simulink model "series_blance_leg"  (R2022b)
settings: Solver=ode45  StartTime=0.0  StopTime=10  MaxStep=0.2  RelTol=1e-3
values from neighbouring files (symbols this model uses):
  a11 = polyfit(leg,k11,3)    [series_get_k.m]
  a12 = polyfit(leg,k12,3)    [series_get_k.m]
  a13 = polyfit(leg,k13,3)    [series_get_k.m]
  a14 = polyfit(leg,k14,3)    [series_get_k.m]
  a15 = polyfit(leg,k15,3)    [series_get_k.m]
  a16 = polyfit(leg,k16,3)    [series_get_k.m]
  a21 = polyfit(leg,k21,3)    [series_get_k.m]
  a22 = polyfit(leg,k22,3)    [series_get_k.m]
  a23 = polyfit(leg,k23,3)    [series_get_k.m]
  a24 = polyfit(leg,k24,3)    [series_get_k.m]
  a25 = polyfit(leg,k25,3)    [series_get_k.m]
  a26 = polyfit(leg,k26,3)    [series_get_k.m]
  N = NM + mp*diff(x + L*sin(theta),t,2)    [series_get_k_length.m]
undefined symbols (not defined in the file or in its folder): X, Y, Z
libraries: sm_lib x60, nesl_utility x20, matrix_library x8, slpidlib x2, cstblocks x2
(part 1 of 3)
settings Model: SimulationMode=accelerator  Creator=Hhop  LastModifiedBy=admin
settings SolverCC: MinimalZcImpactIntegration=on
settings DataIOCC: ReturnWorkspaceOutputs=off
settings DebuggingCC: ReadBeforeWriteMsg=DisableAll  WriteAfterWriteMsg=DisableAll  WriteAfterReadMsg=DisableAll  MultiTaskDSMMsg=none
settings ModelReferenceCC: UpdateModelReferenceTargets=IfOutOfDate
settings SFSimCC: SFSimEcho=off

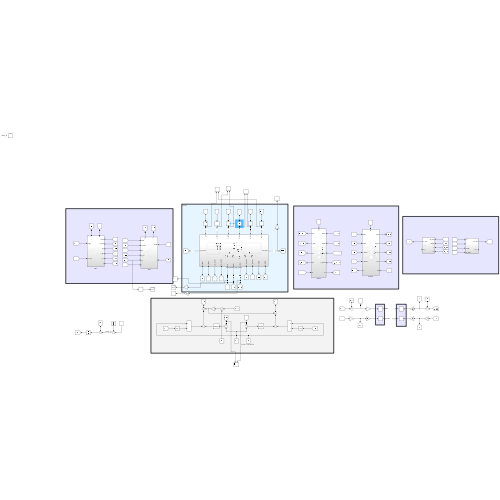
[thumbnail: Simulink's stored preview of the top-level diagram]
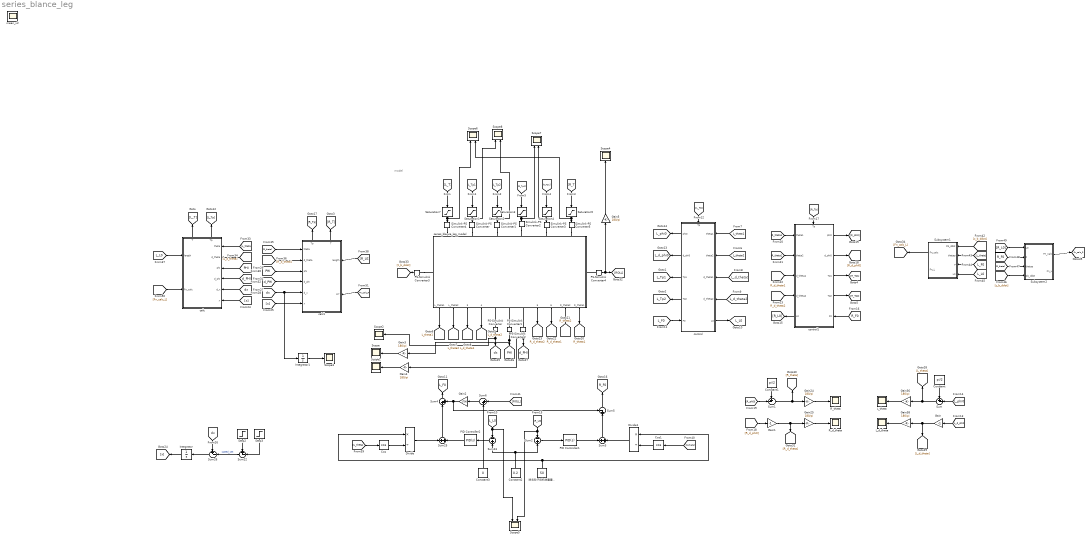
== system series_blance_leg ==
  note: model
  Constant : Constant  Value=pi/2
  Constant1 : Constant  Value=pi/2
  Constant2 : Constant  Value=0.2
  Constant3 : Constant  Value=0
  Cos : Trigonometry  Operator=cos
  Cos1 : Trigonometry  Operator=cos
  Divide : Product  Inputs=*/
  Divide1 : Product  Inputs=*/
  Gain : Gain  Gain=-1
  Gain1 : Gain  Gain=-1
  Gain2 : Gain  Gain=1700
  Gain{3..5,24..25,36,38} (7 alike) : Gain  Gain=180/pi
  Integrator : Integrator
  Integrator1 : Integrator
  L_d_theta : Scope
  L_theta : Scope
  PID Controller1 : slpidlib/PID Controller  Controller=PID  Form=Parallel  TimeDomain=Continuous-time  UseExternalTs=off  SampleTime=-1  IntegratorMethod=Forward Euler  FilterMethod=Forward Euler  ControllerParametersSource=internal  P=800  I=0  UseKiTs=off  D=300  N=100  UseFilter=on  TunerSelectOption=Transfer Function Based (PID Tuner App)  InitialConditionSource=internal  InitialConditionForIntegrator=0  InitialConditionForFilter=0  DifferentiatorICPrevScaledInput=0  ExternalReset=none  TrackingMode=off  Kt=1  LimitOutput=off  SatLimitsSource=internal  UpperSaturationLimit=inf  LowerSaturationLimit=-inf  LinearizeAsGain=on  AntiWindupMode=none  Kb=1  LimitIntegrator=off  UpperIntegratorSaturationLimit=inf  LowerIntegratorSaturationLimit=-inf  POutMin=[]  POutMax=[]  IOutMin=[]  IOutMax=[]  DOutMin=[]  DOutMax=[]  NOutMin=[]  NOutMax=[]  SumOutMin=[]  SumOutMax=[]  SaturationOutMin=[]  SaturationOutMax=[]  PParamMin=[]  PParamMax=[]  IParamMin=[]  IParamMax=[]  DParamMin=[]  DParamMax=[]  NParamMin=[]  NParamMax=[]  KbParamMin=[]  KbParamMax=[]  KtParamMin=[]  KtParamMax=[]  KbOutMin=[]  KbOutMax=[]  KtOutMin=[]  KtOutMax=[]  IntegratorOutMin=[]  IntegratorOutMax=[]  FilterOutMin=[]  FilterOutMax=[]  SumI1OutMin=[]  SumI1OutMax=[]  SumI2OutMin=[]  SumI2OutMax=[]  SumI3OutMin=[]  SumI3OutMax=[]  SumI4OutMin=[]  SumI4OutMax=[]  SumDOutMin=[]  SumDOutMax=[]  DifferentiatorOutMin=[]  DifferentiatorOutMax=[]  FilterDiffOutCoefMin=[]  FilterDiffOutCoefMax=[]  ReciprocalOutMin=[]  ReciprocalOutMax=[]  SumDenOutMin=[]  SumDenOutMax=[]  SumNumOutMin=[]  SumNumOutMax=[]  DivideOutMin=[]  DivideOutMax=[]  UdiffTsProdOutMin=[]  UdiffTsProdOutMax=[]  NTsProdOutMin=[]  NTsProdOutMax=[]  UintegralTsProdOutMin=[]  UintegralTsProdOutMax=[]  UngainTsProdOutMin=[]  UngainTsProdOutMax=[]  ClampingZeroOutDataTypeStr=Inherit: Inherit via back propagation  ClampingZeroOutMin=[]  ClampingZeroOutMax=[]  FilterDenConstantOutDataTypeStr=Inherit: Inherit via back propagation  FilterDenConstantOutMin=[]  FilterDenConstantOutMax=[]  PCopyOutDataTypeStr=Inherit: Inherit via back propagation  PCopyOutMin=[]  PCopyOutMax=[]  NCopyOutDataTypeStr=Inherit: Inherit via back propagation  NCopyOutMin=[]  NCopyOutMax=[]  IntegratorContinuousStateAttributes=''  IntegratorStateMustResolveToSignalObject=off  IntegratorRTWStateStorageClass=Auto  FilterContinuousStateAttributes=''  FilterStateMustResolveToSignalObject=off  FilterRTWStateStorageClass=Auto  ParallelPVariant=InternalParameters  IdealPVariant=Disabled  IVariant=InternalParameters  DVariant=InternalParameters  IntegratorVariant=Continuous  SatVariant=Disabled  AWVariant=Passthrough  PCopyVariant=Disabled  TRVariant=Disabled  FdbkBlocksVariant=Forward  IdealPFdbkVariant=Disabled  SatFdbkVariant=Disabled  DerivativeFilterVariant=ContFilter  NVariant=InternalParameters  NCopyVariant=Disabled  FilterICVariant=InternalICsFilter  IntegratorICVariant=InternalICs  ExternalResetVariant=Disabled  TRSumVariant=Passthrough  SumFdbkVariant=Disabled  SumVariant=Sum_PID  TsampFilterVariant=InternalTs  TsampNgainVariant=Passthrough  TsampIntegralVariant=Passthrough  ExternalSaturationOutDataTypeStr=Inherit: Same as second input
  PID Controller2 : slpidlib/PID Controller  Controller=PID  Form=Parallel  TimeDomain=Continuous-time  UseExternalTs=off  SampleTime=-1  IntegratorMethod=Forward Euler  FilterMethod=Forward Euler  ControllerParametersSource=internal  P=800  I=0  UseKiTs=off  D=300  N=100  UseFilter=on  TunerSelectOption=Transfer Function Based (PID Tuner App)  InitialConditionSource=internal  InitialConditionForIntegrator=0  InitialConditionForFilter=0  DifferentiatorICPrevScaledInput=0  ExternalReset=none  TrackingMode=off  Kt=1  LimitOutput=off  SatLimitsSource=internal  UpperSaturationLimit=inf  LowerSaturationLimit=-inf  LinearizeAsGain=on  AntiWindupMode=none  Kb=1  LimitIntegrator=off  UpperIntegratorSaturationLimit=inf  LowerIntegratorSaturationLimit=-inf  POutMin=[]  POutMax=[]  IOutMin=[]  IOutMax=[]  DOutMin=[]  DOutMax=[]  NOutMin=[]  NOutMax=[]  SumOutMin=[]  SumOutMax=[]  SaturationOutMin=[]  SaturationOutMax=[]  PParamMin=[]  PParamMax=[]  IParamMin=[]  IParamMax=[]  DParamMin=[]  DParamMax=[]  NParamMin=[]  NParamMax=[]  KbParamMin=[]  KbParamMax=[]  KtParamMin=[]  KtParamMax=[]  KbOutMin=[]  KbOutMax=[]  KtOutMin=[]  KtOutMax=[]  IntegratorOutMin=[]  IntegratorOutMax=[]  FilterOutMin=[]  FilterOutMax=[]  SumI1OutMin=[]  SumI1OutMax=[]  SumI2OutMin=[]  SumI2OutMax=[]  SumI3OutMin=[]  SumI3OutMax=[]  SumI4OutMin=[]  SumI4OutMax=[]  SumDOutMin=[]  SumDOutMax=[]  DifferentiatorOutMin=[]  DifferentiatorOutMax=[]  FilterDiffOutCoefMin=[]  FilterDiffOutCoefMax=[]  ReciprocalOutMin=[]  ReciprocalOutMax=[]  SumDenOutMin=[]  SumDenOutMax=[]  SumNumOutMin=[]  SumNumOutMax=[]  DivideOutMin=[]  DivideOutMax=[]  UdiffTsProdOutMin=[]  UdiffTsProdOutMax=[]  NTsProdOutMin=[]  NTsProdOutMax=[]  UintegralTsProdOutMin=[]  UintegralTsProdOutMax=[]  UngainTsProdOutMin=[]  UngainTsProdOutMax=[]  ClampingZeroOutDataTypeStr=Inherit: Inherit via back propagation  ClampingZeroOutMin=[]  ClampingZeroOutMax=[]  FilterDenConstantOutDataTypeStr=Inherit: Inherit via back propagation  FilterDenConstantOutMin=[]  FilterDenConstantOutMax=[]  PCopyOutDataTypeStr=Inherit: Inherit via back propagation  PCopyOutMin=[]  PCopyOutMax=[]  NCopyOutDataTypeStr=Inherit: Inherit via back propagation  NCopyOutMin=[]  NCopyOutMax=[]  IntegratorContinuousStateAttributes=''  IntegratorStateMustResolveToSignalObject=off  IntegratorRTWStateStorageClass=Auto  FilterContinuousStateAttributes=''  FilterStateMustResolveToSignalObject=off  FilterRTWStateStorageClass=Auto  ParallelPVariant=InternalParameters  IdealPVariant=Disabled  IVariant=InternalParameters  DVariant=InternalParameters  IntegratorVariant=Continuous  SatVariant=Disabled  AWVariant=Passthrough  PCopyVariant=Disabled  TRVariant=Disabled  FdbkBlocksVariant=Forward  IdealPFdbkVariant=Disabled  SatFdbkVariant=Disabled  DerivativeFilterVariant=ContFilter  NVariant=InternalParameters  NCopyVariant=Disabled  FilterICVariant=InternalICsFilter  IntegratorICVariant=InternalICs  ExternalResetVariant=Disabled  TRSumVariant=Passthrough  SumFdbkVariant=Disabled  SumVariant=Sum_PID  TsampFilterVariant=InternalTs  TsampNgainVariant=Passthrough  TsampIntegralVariant=Passthrough  ExternalSaturationOutDataTypeStr=Inherit: Same as second input
  PS-Simulink Converter{,1..4} (5 alike) : nesl_utility/PS-Simulink Converter  PhysicalDomain=network_engine_domain  SubClassName=ps_output  LeftPortType=input  RightPortType=output  PseudoPeriodic=off  Frequencies=[]  VectorFormat=inherit  Unit=inherit  AffineConversion=off
  R_d_theta : Scope
  R_theta : Scope
  Saturation1 : Saturate  UpperLimit=5  LowerLimit=-5
  Saturation2 : Saturate  UpperLimit=10  LowerLimit=-10
  Saturation3 : Saturate  UpperLimit=10  LowerLimit=-10
  Saturation4 : Saturate  UpperLimit=5  LowerLimit=-5
  Saturation5 : Saturate  UpperLimit=9  LowerLimit=-9
  Saturation7 : Saturate  UpperLimit=9  LowerLimit=-9
  Scope{,1..4} (5 alike) : Scope
  Scope{5..8} (4 alike) : Scope  NumInputPorts=2
  Simulink-PS Converter{,1..5} (6 alike) : nesl_utility/Simulink-PS Converter  PhysicalDomain=network_engine_domain  SubClassName=ps_input  LeftPortType=input  RightPortType=output  PseudoPeriodic=off  Frequencies=[]  NoiseDistribution=none  NoiseParameters=[]  Unit=1  AffineConversion=off  FilteringAndDerivatives=provide  SimscapeFilterOrder=1  InputFilterTimeConstant=0.001  UdotUserProvided=0
  Step2 : Step  After=2.5  SampleTime=0
  Step3 : Step  Time=4.5  After=2.5  SampleTime=0
  Subsystem1 : Subsystem
  Subsystem2 : Subsystem
  Sum{,1,22,26} (4 alike) : Sum  Inputs=+-|
  Sum2 : Sum  Inputs=-|+
  Sum23 : Sum  Inputs=-|+
  Sum25 : Sum  Inputs=+|+
  Sum3 : Sum  Inputs=+|+
  Sum4 : Sum  Inputs=|++
  Sum5 : Sum  Inputs=-+|
  Sum6 : Sum  Inputs=|++
  calc : Subsystem
      settings: PortSchema="{\"entries\":[{\"content\":{\"sides\":[{\"content\":{\"connectorIds\":[\"In1\",\"In2\",\"In3\",\"In4\",\"In5\",\"In6\"]},\"type\":\"ConnectorPlacement.EquallySpacedRectSide\",\"uuid\":\"055cb80c-cd03-4a8d-aef8-6b3df8c72d3f\"},{\"content\":{\"connectorIds\":[\"In7\",\"In8\"],\"side\":\"RIGHT\"},\"type\":\"ConnectorPlacement.EquallySpacedRectSide\",\"uuid\":\"5756fad1-d70f-4a11-a5af-d2f67bfb0d7e\"},{\"content\":{\"connectorIds\":[\"Out1\",\"Out2\"],\"side\":\"TOP\"},\"type\":\"ConnectorPlacement.EquallySpacedRectSide\",\"uuid\":\"9c70cf42-10f8-4525-9406-562484abf580\"},{\"content\":{\"connectorIds\":[],\"side\":\"BOTTOM\"},\"type\":\"ConnectorPlacement.EquallySpacedRectSide\",\"uuid\":\"af43612d-13e3-4981-866d-f85b70daa608\"}]},\"type\":\"ConnectorPlacement.EquallySpacedConnector\",\"uuid\":\"7084d402-0e44-4d2f-8cc2-1336d196e84d\"}],\"packageUris\":[\"http://schema.mathworks.com/mf0/Connector/R2020b\"],\"version\":\"1.0\"}"
  calc1 : Subsystem
      settings: PortSchema="{\"entries\":[{\"content\":{\"sides\":[{\"content\":{\"connectorIds\":[\"In1\",\"In2\",\"In3\",\"In4\",\"In5\",\"In6\"]},\"type\":\"ConnectorPlacement.EquallySpacedRectSide\",\"uuid\":\"055cb80c-cd03-4a8d-aef8-6b3df8c72d3f\"},{\"content\":{\"connectorIds\":[\"In7\",\"In8\"],\"side\":\"RIGHT\"},\"type\":\"ConnectorPlacement.EquallySpacedRectSide\",\"uuid\":\"5756fad1-d70f-4a11-a5af-d2f67bfb0d7e\"},{\"content\":{\"connectorIds\":[],\"side\":\"TOP\"},\"type\":\"ConnectorPlacement.EquallySpacedRectSide\",\"uuid\":\"9c70cf42-10f8-4525-9406-562484abf580\"},{\"content\":{\"connectorIds\":[\"Out1\",\"Out2\"],\"side\":\"BOTTOM\"},\"type\":\"ConnectorPlacement.EquallySpacedRectSide\",\"uuid\":\"965870e0-1376-434b-943d-1e2aec9ec9a4\"}]},\"type\":\"ConnectorPlacement.EquallySpacedConnector\",\"uuid\":\"7084d402-0e44-4d2f-8cc2-1336d196e84d\"}],\"packageUris\":[\"http://schema.mathworks.com/mf0/Connector/R2020b\"],\"version\":\"1.0\"}"
  control : Subsystem
      settings: PortSchema="{\"entries\":[{\"content\":{\"sides\":[{\"content\":{\"connectorIds\":[\"In1\",\"In2\",\"In3\",\"In4\",\"Out5\"]},\"type\":\"ConnectorPlacement.EquallySpacedRectSide\",\"uuid\":\"b67c5c15-541a-42c2-ad41-63265a09e0f2\"},{\"content\":{\"connectorIds\":[\"Out1\",\"Out2\",\"Out3\",\"Out4\",\"In6\"],\"side\":\"RIGHT\"},\"type\":\"ConnectorPlacement.EquallySpacedRectSide\",\"uuid\":\"07f76f3c-6592-43b8-b38c-8fe88f245cee\"},{\"content\":{\"connectorIds\":[\"In5\"],\"side\":\"TOP\"},\"type\":\"ConnectorPlacement.EquallySpacedRectSide\",\"uuid\":\"70cf3606-9c74-4702-8d81-357957bb1572\"}]},\"type\":\"ConnectorPlacement.EquallySpacedConnector\",\"uuid\":\"a816ba83-22f4-422c-bb6b-6512d42bfdf3\"}],\"packageUris\":[\"http://schema.mathworks.com/mf0/Connector/R2020b\"],\"version\":\"1.0\"}"
  control1 : Subsystem
      settings: PortSchema="{\"entries\":[{\"content\":{\"sides\":[{\"content\":{\"connectorIds\":[\"In1\",\"In2\",\"In3\",\"In4\",\"Out5\"]},\"type\":\"ConnectorPlacement.EquallySpacedRectSide\",\"uuid\":\"b67c5c15-541a-42c2-ad41-63265a09e0f2\"},{\"content\":{\"connectorIds\":[\"Out1\",\"Out2\",\"Out3\",\"Out4\",\"In6\"],\"side\":\"RIGHT\"},\"type\":\"ConnectorPlacement.EquallySpacedRectSide\",\"uuid\":\"07f76f3c-6592-43b8-b38c-8fe88f245cee\"},{\"content\":{\"connectorIds\":[\"In5\"],\"side\":\"TOP\"},\"type\":\"ConnectorPlacement.EquallySpacedRectSide\",\"uuid\":\"70cf3606-9c74-4702-8d81-357957bb1572\"}]},\"type\":\"ConnectorPlacement.EquallySpacedConnector\",\"uuid\":\"a816ba83-22f4-422c-bb6b-6512d42bfdf3\"}],\"packageUris\":[\"http://schema.mathworks.com/mf0/Connector/R2020b\"],\"version\":\"1.0\"}"
  mean_x2 : Scope
  series_blance_leg_model : Subsystem
      settings: PortSchema="{\"entries\":[{\"content\":{\"sides\":[{\"content\":{\"connectorIds\":[\"LConn1\",\"LConn2\",\"LConn3\",\"LConn4\",\"LConn5\",\"LConn6\"]},\"type\":\"ConnectorPlacement.EquallySpacedRectSide\",\"uuid\":\"ed635f35-0836-4900-93e3-56fc3520c8de\"},{\"content\":{\"connectorIds\":[\"Out1\",\"Out2\",\"Out3\",\"Out4\",\"RConn1\",\"RConn2\",\"RConn3\",\"Out5\",\"Out6\",\"Out7\",\"Out8\"],\"side\":\"RIGHT\"},\"type\":\"ConnectorPlacement.EquallySpacedRectSide\",\"uuid\":\"bb235ec0-defd-4ad9-96f6-8533dab3fbd9\"},{\"content\":{\"connectorIds\":[\"LConn7\"],\"side\":\"TOP\"},\"type\":\"ConnectorPlacement.EquallySpacedRectSide\",\"uuid\":\"d719db37-8b3a-4344-b330-944fde418334\"},{\"content\":{\"connectorIds\":[\"RConn4\"],\"side\":\"BOTTOM\"},\"type\":\"ConnectorPlacement.EquallySpacedRectSide\",\"uuid\":\"20f9270b-6ab1-4e89-bf00-e838d12c3c13\"}]},\"type\":\"ConnectorPlacement.EquallySpacedConnector\",\"uuid\":\"a2f25b71-0047-4a2d-a238-dad76f034ab1\"}],\"packageUris\":[\"http://schema.mathworks.com/mf0/Connector/R2020b\"],\"version\":\"1.0\"}"
  除去轮子后机体重量， : Constant  Value=50
  tag scope: Fn_calc_R=global, L_F0=global, L_L0=global, L_Tp1=global, L_Tp2=global, L_d_phi0=global, L_d_theta1=global, L_d_theta2=global, L_phi0=global, L_theta1=global, L_theta2=global, PHI=global, R_F0=global, R_d_theta1=global, R_d_theta2=global, R_theta1=global, R_theta2=global, d_PHI=global, dx=global
  wires:
  Gain36/1 -> L_theta/1
  Gain38/1 -> L_d_theta/1
  Gain/1 -> [L_d_theta], Gain38/1
  Sum/1 -> [L_theta], Gain36/1
  Constant/1 -> Sum/1
  Gain25/1 -> R_d_theta/1
  Gain24/1 -> R_theta/1
  Sum1/1 -> [R_theta], Gain24/1
  Constant1/1 -> Sum1/1
  Gain1/1 -> [R_d_theta], Gain25/1
  PID Controller2/1 -> Sum25/2
  除去轮子后机体重量，/1 -> Divide1/1, Divide/1
  Sum23/1 -> PID Controller2/1
  Constant2/1 -> Sum2/2, Sum23/2
  Sum2/1 -> PID Controller1/1
  PID Controller1/1 -> Sum3/1
  Step3/1 -> Sum22/2
  Sum26/1 -> Integrator/1
  Step2/1 -> Sum22/1
  Sum22/1 -> Sum26/2  "speed_set"
  Saturation7/1 -> Scope6/1, Simulink-PS Converter4/1
  Saturation1/1 -> Scope8/1, Simulink-PS Converter/1
  Saturation2/1 -> Scope8/2, Simulink-PS Converter1/1
  Saturation3/1 -> Scope7/1, Simulink-PS Converter2/1
  Saturation4/1 -> Scope7/2, Simulink-PS Converter3/1
  Saturation5/1 -> Scope6/2, Simulink-PS Converter5/1
  calc/2(T) -> [L_T]
  [L_T] -> Saturation7/1
  control/3(Tp1) -> [L_Tp1]
  [L_Tp1] -> Saturation1/1
  control/4(Tp2) -> [L_Tp2]
  [L_Tp2] -> Saturation2/1
  calc1/2(T) -> [R_T]
  [R_T] -> Saturation5/1
  control1/3(Tp1) -> [R_Tp1]
  [R_Tp1] -> Saturation4/1
  control1/4(Tp2) -> [R_Tp2]
  [R_Tp2] -> Saturation3/1
  series_blance_leg_model/1(L_theta1) -> [L_theta1]
  [L_theta1] -> control/1(theta1)
  series_blance_leg_model/2(L_theta2) -> [L_theta2]
  [L_theta2] -> control/2(theta2)
  series_blance_leg_model/3(L_d_theta1) -> [L_d_theta1]
  [L_d_theta1] -> control/3(d_theta1)
  series_blance_leg_model/4(L_d_theta2) -> [L_d_theta2]
  [L_d_theta2] -> control/4(d_theta2)
  control/5(L0) -> [L_L0]
  [L_L0] -> Scope5/1, Sum23/1
  [L_F0] -> control/6(F0)
  calc/1(Tp) -> [L_Tp]
  [L_Tp] -> control/5(Tp)
  control/2(d_phi0) -> [L_d_phi0]
  [L_d_phi0] -> Gain/1
  control/1(phi0) -> [L_phi0]
  [L_phi0] -> Sum/2
  control1/5(L0) -> [R_L0]
  [R_L0] -> Scope5/2, Sum2/1
  [R_F0] -> control1/6(F0)
  [R_Tp] -> control1/5(Tp)
  calc1/1(Tp) -> [R_Tp]
  control1/2(d_phi0) -> [R_d_phi0]
  [R_d_phi0] -> Gain1/1
  control1/1(phi0) -> [R_phi0]
  [R_phi0] -> Sum1/2
  series_blance_leg_model/8(R_theta1) -> [R_theta1]
  [R_theta1] -> control1/1(theta1)
  series_blance_leg_model/7(R_theta2) -> [R_theta2]
  [R_theta2] -> control1/2(theta2)
  series_blance_leg_model/6(R_d_theta1) -> [R_d_theta1]
  [R_d_theta1] -> control1/3(d_theta1)
  series_blance_leg_model/5(R_d_theta2) -> [R_d_theta2]
  [R_d_theta2] -> control1/4(d_theta2)
  [x] -> calc/6(x)
  [x] -> calc1/1(x)
  Integrator/1 -> [x]
  [dx] -> Sum26/1
  [dx] -> calc/5(d_x)
  PS-Simulink Converter/1 -> Scope2/1, [dx]
  [dx] -> Integrator1/1, calc1/2(d_x)
  PS-Simulink Converter1/1 -> Gain3/1, [PHI]
  [PHI] -> calc/3(phi)
  [PHI] -> calc1/4(phi)
  PS-Simulink Converter2/1 -> Gain4/1, [d_PHI]
  [d_PHI] -> calc/4(d_phi)
  [d_PHI] -> calc1/3(d_phi)
  [L_theta] -> calc/1(theta)
  [L_d_theta] -> calc/2(d_theta)
  [R_theta] -> calc1/6(theta)
  [R_d_theta] -> calc1/5(d_theta)
  [L_L0] -> calc/7(length)
  [R_L0] -> calc1/8(length)
  Divide/1 -> Sum25/1
  Cos/1 -> Divide/2
  [L_theta] -> Cos/1
  Cos1/1 -> Divide1/2
  Divide1/1 -> Sum3/2
  [R_theta] -> Cos1/1
  Sum4/1 -> [L_F0]
  Sum25/1 -> Sum4/1
  Sum5/1 -> [R_F0]
  Sum3/1 -> Sum5/2
  Sum6/1 -> Gain2/1
  Constant3/1 -> Sum6/2
  Gain2/1 -> Sum5/1, Sum4/2
  PS-Simulink Converter4/1 -> [ROLL], Gain5/1
  [ROLL] -> Sum6/1
  PS-Simulink Converter3/1 -> [z_b_ddot]
  [z_b_ddot] -> Subsystem1/1(Zb_ddot)
  [L_theta] -> Subsystem1/2(thetap)
  [L_F0] -> Subsystem1/3(F)
  [L_L0] -> Subsystem1/4(L0)
  [R_theta] -> Subsystem2/2(thetap)
  [z_b_ddot] -> Subsystem2/1(Zb_ddot)
  [R_L0] -> Subsystem2/4(L0)
  [R_F0] -> Subsystem2/3(F)
  [Fn_calc_L] -> calc/8(Fn_calc)
  Subsystem1/1(Fn_calc) -> [Fn_calc_L]
  [Fn_calc_R] -> calc1/7(In7)
  Subsystem2/2(Fn_calc) -> [Fn_calc_R]
  Gain3/1 -> Scope/1
  Gain4/1 -> Scope1/1
  Gain5/1 -> Scope4/1
  Integrator1/1 -> Scope3/1
  connections:
  PS-Simulink Converter/LConn1 -- series_blance_leg_model/RConn1
  PS-Simulink Converter1/LConn1 -- series_blance_leg_model/RConn2
  PS-Simulink Converter2/LConn1 -- series_blance_leg_model/RConn3
  Simulink-PS Converter/RConn1 -- series_blance_leg_model/LConn2
  Simulink-PS Converter1/RConn1 -- series_blance_leg_model/LConn3
  Simulink-PS Converter3/RConn1 -- series_blance_leg_model/LConn5
  Simulink-PS Converter2/RConn1 -- series_blance_leg_model/LConn4
  Simulink-PS Converter4/RConn1 -- series_blance_leg_model/LConn1
  Simulink-PS Converter5/RConn1 -- series_blance_leg_model/LConn6
  PS-Simulink Converter3/LConn1 -- series_blance_leg_model/LConn7
  PS-Simulink Converter4/LConn1 -- series_blance_leg_model/RConn4

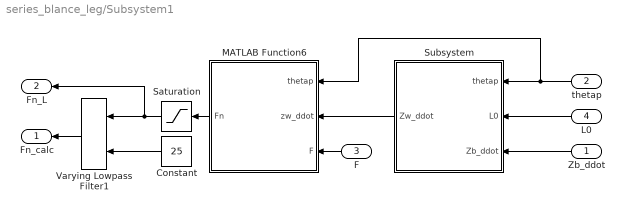
== system series_blance_leg/Subsystem1 ==
  Zb_ddot : Inport
  thetap : Inport  Port=2
  F : Inport  Port=3
  L0 : Inport  Port=4
  Constant : Constant  Value=25
  MATLAB Function6 : MATLAB Function  TreatAsAtomicUnit=on
  Saturation : Saturate  UpperLimit=120  LowerLimit=-20  ZeroCross=off
  Subsystem : Subsystem
  Varying Lowpass Filter1 : cstblocks/Linear Parameter Varying/Varying Lowpass Filter  N=2
  Fn_calc : Outport
  Fn_L : Outport  Port=2
  wires:
  Subsystem/1(Zw_ddot) -> MATLAB Function6/2(zw_ddot)
  thetap/1 -> MATLAB Function6/1(thetap), Subsystem/1(thetap)
  F/1 -> MATLAB Function6/3(F)
  Zb_ddot/1 -> Subsystem/3(Zb_ddot)
  L0/1 -> Subsystem/2(L0)
  Constant/1 -> Varying Lowpass Filter1/2
  Saturation/1 -> Fn_L/1, Varying Lowpass Filter1/1
  Varying Lowpass Filter1/1 -> Fn_calc/1
  MATLAB Function6/1(Fn) -> Saturation/1

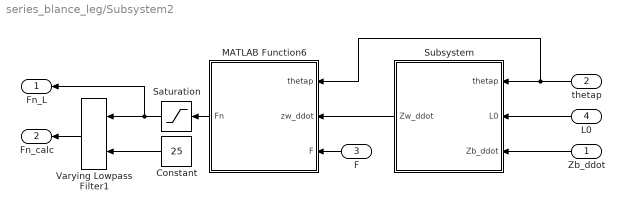
== system series_blance_leg/Subsystem2 ==
  Zb_ddot : Inport
  thetap : Inport  Port=2
  F : Inport  Port=3
  L0 : Inport  Port=4
  Constant : Constant  Value=25
  MATLAB Function6 : MATLAB Function  TreatAsAtomicUnit=on
  Saturation : Saturate  UpperLimit=120  LowerLimit=-20  ZeroCross=off
  Subsystem : Subsystem
  Varying Lowpass Filter1 : cstblocks/Linear Parameter Varying/Varying Lowpass Filter  N=2
  Fn_L : Outport
  Fn_calc : Outport  Port=2
  wires:
  Subsystem/1(Zw_ddot) -> MATLAB Function6/2(zw_ddot)
  thetap/1 -> MATLAB Function6/1(thetap), Subsystem/1(thetap)
  F/1 -> MATLAB Function6/3(F)
  Zb_ddot/1 -> Subsystem/3(Zb_ddot)
  L0/1 -> Subsystem/2(L0)
  Constant/1 -> Varying Lowpass Filter1/2
  Saturation/1 -> Fn_L/1, Varying Lowpass Filter1/1
  Varying Lowpass Filter1/1 -> Fn_calc/1
  MATLAB Function6/1(Fn) -> Saturation/1

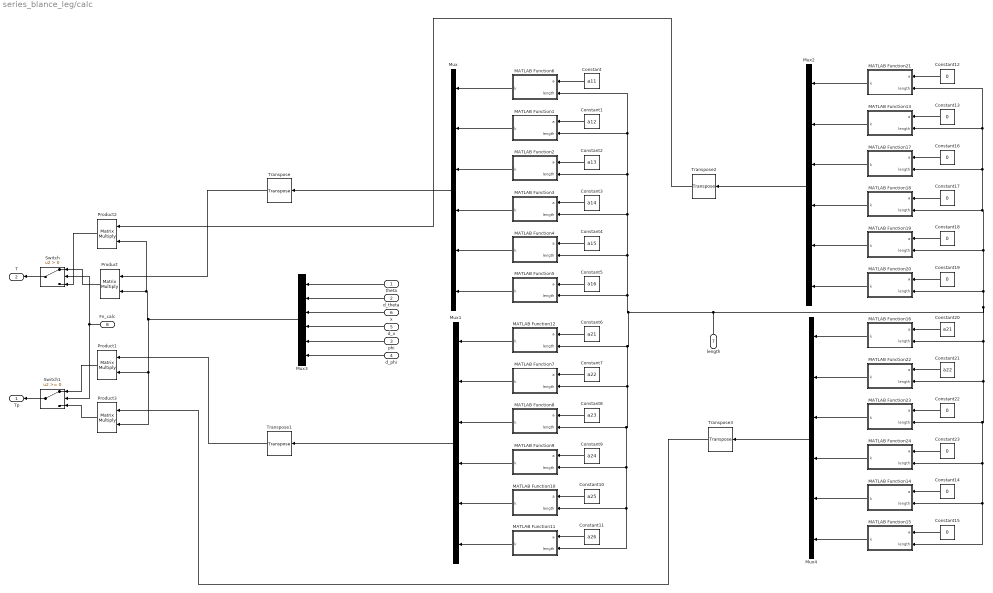
== system series_blance_leg/calc ==
  theta : Inport
  d_theta : Inport  Port=2
  phi : Inport  Port=3
  d_phi : Inport  Port=4
  d_x : Inport  Port=5
  x : Inport  Port=6
  length : Inport  Port=7
  Fn_calc : Inport  Port=8
  Constant : Constant  Value=a11
  Constant1 : Constant  Value=a12
  Constant10 : Constant  Value=a25
  Constant11 : Constant  Value=a26
  Constant{12..19,22..23} (10 alike) : Constant  Value=0
  Constant2 : Constant  Value=a13
  Constant20 : Constant  Value=a21
  Constant21 : Constant  Value=a22
  Constant3 : Constant  Value=a14
  Constant4 : Constant  Value=a15
  Constant5 : Constant  Value=a16
  Constant6 : Constant  Value=a21
  Constant7 : Constant  Value=a22
  Constant8 : Constant  Value=a23
  Constant9 : Constant  Value=a24
  MATLAB Function1 : MATLAB Function  TreatAsAtomicUnit=on
  MATLAB Function10 : MATLAB Function  TreatAsAtomicUnit=on
  MATLAB Function11 : MATLAB Function  TreatAsAtomicUnit=on
  MATLAB Function12 : MATLAB Function  TreatAsAtomicUnit=on
  MATLAB Function13 : MATLAB Function  TreatAsAtomicUnit=on
  MATLAB Function14 : MATLAB Function  TreatAsAtomicUnit=on
  MATLAB Function15 : MATLAB Function  TreatAsAtomicUnit=on
  MATLAB Function16 : MATLAB Function  TreatAsAtomicUnit=on
  MATLAB Function17 : MATLAB Function  TreatAsAtomicUnit=on
  MATLAB Function18 : MATLAB Function  TreatAsAtomicUnit=on
  MATLAB Function19 : MATLAB Function  TreatAsAtomicUnit=on
  MATLAB Function2 : MATLAB Function  TreatAsAtomicUnit=on
  MATLAB Function20 : MATLAB Function  TreatAsAtomicUnit=on
  MATLAB Function21 : MATLAB Function  TreatAsAtomicUnit=on
  MATLAB Function22 : MATLAB Function  TreatAsAtomicUnit=on
  MATLAB Function23 : MATLAB Function  TreatAsAtomicUnit=on
  MATLAB Function24 : MATLAB Function  TreatAsAtomicUnit=on
  MATLAB Function3 : MATLAB Function  TreatAsAtomicUnit=on
  MATLAB Function4 : MATLAB Function  TreatAsAtomicUnit=on
  MATLAB Function5 : MATLAB Function  TreatAsAtomicUnit=on
  MATLAB Function6 : MATLAB Function  TreatAsAtomicUnit=on
  MATLAB Function7 : MATLAB Function  TreatAsAtomicUnit=on
  MATLAB Function8 : MATLAB Function  TreatAsAtomicUnit=on
  MATLAB Function9 : MATLAB Function  TreatAsAtomicUnit=on
  Mux{,1..4} (5 alike) : Mux  Inputs=6
  Product{,1..3} (4 alike) : Product  Multiplication=Matrix(*)
  Switch : Switch  Criteria=u2 > Threshold  ZeroCross=off  SaturateOnIntegerOverflow=off  InputSameDT=off
  Switch1 : Switch  ZeroCross=off  SaturateOnIntegerOverflow=off  InputSameDT=off
  Transpose{,1..3} (4 alike) : matrix_library/Transpose
  Tp : Outport
  T : Outport  Port=2
  wires:
  theta/1 -> Mux3/1
  d_theta/1 -> Mux3/2
  x/1 -> Mux3/3
  d_x/1 -> Mux3/4
  phi/1 -> Mux3/5
  d_phi/1 -> Mux3/6
  Mux/1 -> Transpose/1
  Constant5/1 -> MATLAB Function5/1(a)
  MATLAB Function6/1(k) -> Mux/1
  MATLAB Function3/1(k) -> Mux/4
  Constant9/1 -> MATLAB Function9/1(a)
  Constant7/1 -> MATLAB Function7/1(a)
  MATLAB Function2/1(k) -> Mux/3
  MATLAB Function1/1(k) -> Mux/2
  Constant4/1 -> MATLAB Function4/1(a)
  MATLAB Function12/1(k) -> Mux1/1
  Constant/1 -> MATLAB Function6/1(a)
  MATLAB Function9/1(k) -> Mux1/4
  MATLAB Function8/1(k) -> Mux1/3
  Constant6/1 -> MATLAB Function12/1(a)
  Constant1/1 -> MATLAB Function1/1(a)
  Constant8/1 -> MATLAB Function8/1(a)
  Constant3/1 -> MATLAB Function3/1(a)
  Constant2/1 -> MATLAB Function2/1(a)
  MATLAB Function5/1(k) -> Mux/6
  MATLAB Function4/1(k) -> Mux/5
  MATLAB Function11/1(k) -> Mux1/6
  Constant11/1 -> MATLAB Function11/1(a)
  MATLAB Function10/1(k) -> Mux1/5
  Mux1/1 -> Transpose1/1
  MATLAB Function7/1(k) -> Mux1/2
  Constant10/1 -> MATLAB Function10/1(a)
  Transpose/1 -> Product/1
  Mux3/1 -> Product1/2, Product3/2, Product2/2, Product/2
  Transpose1/1 -> Product1/1
  Mux4/1 -> Transpose3/1
  MATLAB Function16/1(k) -> Mux4/1
  Constant15/1 -> MATLAB Function15/1(a)
  MATLAB Function15/1(k) -> Mux4/6
  MATLAB Function20/1(k) -> Mux2/6
  Constant16/1 -> MATLAB Function17/1(a)
  MATLAB Function19/1(k) -> Mux2/5
  Constant20/1 -> MATLAB Function16/1(a)
  MATLAB Function23/1(k) -> Mux4/3
  MATLAB Function24/1(k) -> Mux4/4
  MATLAB Function21/1(k) -> Mux2/1
  length/1 -> MATLAB Function9/2(length), MATLAB Function10/2(length), MATLAB Function11/2(length), MATLAB Function8/2(length), MATLAB Function7/2(length), MATLAB Function12/2(length), MATLAB Function6/2(length), MATLAB Function1/2(length), MATLAB Function2/2(length), MATLAB Function3/2(length), MATLAB Function4/2(length), MATLAB Function5/2(length), MATLAB Function24/2(length), MATLAB Function14/2(length), MATLAB Function15/2(length), MATLAB Function23/2(length), MATLAB Function22/2(length), MATLAB Function16/2(length), MATLAB Function21/2(length), MATLAB Function13/2(length), MATLAB Function17/2(length), MATLAB Function18/2(length), MATLAB Function19/2(length), MATLAB Function20/2(length)
  Constant23/1 -> MATLAB Function24/1(a)
  Constant21/1 -> MATLAB Function22/1(a)
  Constant18/1 -> MATLAB Function19/1(a)
  Constant19/1 -> MATLAB Function20/1(a)
  Constant17/1 -> MATLAB Function18/1(a)
  Constant22/1 -> MATLAB Function23/1(a)
  Constant13/1 -> MATLAB Function13/1(a)
  Constant14/1 -> MATLAB Function14/1(a)
  MATLAB Function14/1(k) -> Mux4/5
  MATLAB Function22/1(k) -> Mux4/2
  MATLAB Function13/1(k) -> Mux2/2
  MATLAB Function17/1(k) -> Mux2/3
  MATLAB Function18/1(k) -> Mux2/4
  Mux2/1 -> Transpose2/1
  Constant12/1 -> MATLAB Function21/1(a)
  Transpose2/1 -> Product2/1
  Transpose3/1 -> Product3/1
  Product/1 -> Switch/1
  Product2/1 -> Switch/3
  Switch/1 -> T/1
  Product1/1 -> Switch1/1
  Product3/1 -> Switch1/3
  Switch1/1 -> Tp/1
  Fn_calc/1 -> Switch1/2, Switch/2

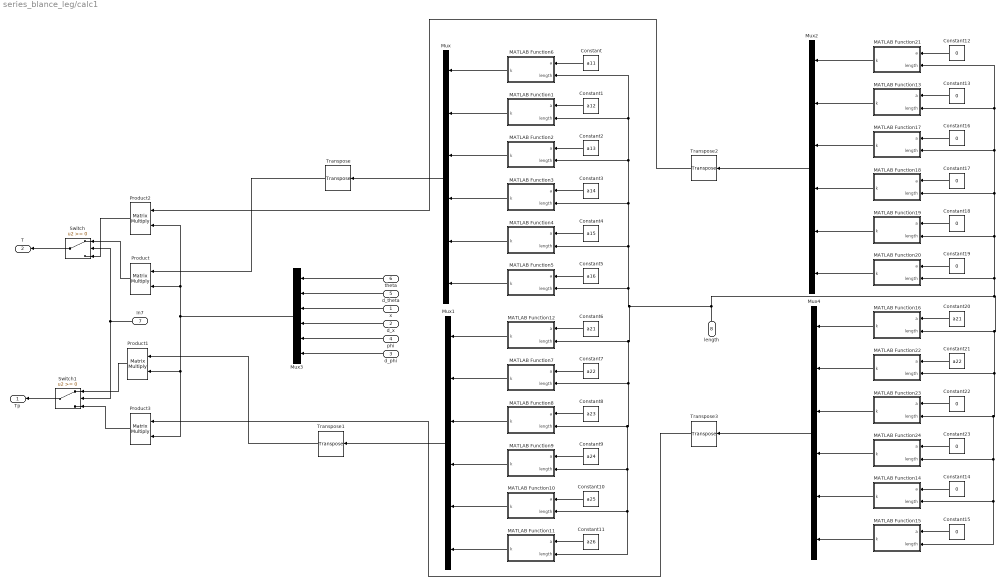
== system series_blance_leg/calc1 ==
  x : Inport
  d_x : Inport  Port=2
  d_phi : Inport  Port=3
  phi : Inport  Port=4
  d_theta : Inport  Port=5
  theta : Inport  Port=6
  In7 : Inport  Port=7
  length : Inport  Port=8
  Constant : Constant  Value=a11
  Constant1 : Constant  Value=a12
  Constant10 : Constant  Value=a25
  Constant11 : Constant  Value=a26
  Constant{12..19,22..23} (10 alike) : Constant  Value=0
  Constant2 : Constant  Value=a13
  Constant20 : Constant  Value=a21
  Constant21 : Constant  Value=a22
  Constant3 : Constant  Value=a14
  Constant4 : Constant  Value=a15
  Constant5 : Constant  Value=a16
  Constant6 : Constant  Value=a21
  Constant7 : Constant  Value=a22
  Constant8 : Constant  Value=a23
  Constant9 : Constant  Value=a24
  MATLAB Function1 : MATLAB Function  TreatAsAtomicUnit=on
  MATLAB Function10 : MATLAB Function  TreatAsAtomicUnit=on
  MATLAB Function11 : MATLAB Function  TreatAsAtomicUnit=on
  MATLAB Function12 : MATLAB Function  TreatAsAtomicUnit=on
  MATLAB Function13 : MATLAB Function  TreatAsAtomicUnit=on
  MATLAB Function14 : MATLAB Function  TreatAsAtomicUnit=on
  MATLAB Function15 : MATLAB Function  TreatAsAtomicUnit=on
  MATLAB Function16 : MATLAB Function  TreatAsAtomicUnit=on
  MATLAB Function17 : MATLAB Function  TreatAsAtomicUnit=on
  MATLAB Function18 : MATLAB Function  TreatAsAtomicUnit=on
  MATLAB Function19 : MATLAB Function  TreatAsAtomicUnit=on
  MATLAB Function2 : MATLAB Function  TreatAsAtomicUnit=on
  MATLAB Function20 : MATLAB Function  TreatAsAtomicUnit=on
  MATLAB Function21 : MATLAB Function  TreatAsAtomicUnit=on
  MATLAB Function22 : MATLAB Function  TreatAsAtomicUnit=on
  MATLAB Function23 : MATLAB Function  TreatAsAtomicUnit=on
  MATLAB Function24 : MATLAB Function  TreatAsAtomicUnit=on
  MATLAB Function3 : MATLAB Function  TreatAsAtomicUnit=on
  MATLAB Function4 : MATLAB Function  TreatAsAtomicUnit=on
  MATLAB Function5 : MATLAB Function  TreatAsAtomicUnit=on
  MATLAB Function6 : MATLAB Function  TreatAsAtomicUnit=on
  MATLAB Function7 : MATLAB Function  TreatAsAtomicUnit=on
  MATLAB Function8 : MATLAB Function  TreatAsAtomicUnit=on
  MATLAB Function9 : MATLAB Function  TreatAsAtomicUnit=on
  Mux{,1..4} (5 alike) : Mux  Inputs=6
  Product{,1..3} (4 alike) : Product  Multiplication=Matrix(*)
  Switch : Switch  ZeroCross=off  SaturateOnIntegerOverflow=off  InputSameDT=off
  Switch1 : Switch  ZeroCross=off  SaturateOnIntegerOverflow=off  InputSameDT=off
  Transpose{,1..3} (4 alike) : matrix_library/Transpose
  Tp : Outport
  T : Outport  Port=2
  wires:
  d_phi/1 -> Mux3/6
  phi/1 -> Mux3/5
  d_x/1 -> Mux3/4
  x/1 -> Mux3/3
  d_theta/1 -> Mux3/2
  theta/1 -> Mux3/1
  Mux/1 -> Transpose/1
  Mux3/1 -> Product3/2, Product1/2, Product2/2, Product/2
  Mux1/1 -> Transpose1/1
  Constant5/1 -> MATLAB Function5/1(a)
  MATLAB Function6/1(k) -> Mux/1
  MATLAB Function3/1(k) -> Mux/4
  Constant9/1 -> MATLAB Function9/1(a)
  Constant7/1 -> MATLAB Function7/1(a)
  MATLAB Function2/1(k) -> Mux/3
  MATLAB Function1/1(k) -> Mux/2
  Constant4/1 -> MATLAB Function4/1(a)
  MATLAB Function12/1(k) -> Mux1/1
  Constant/1 -> MATLAB Function6/1(a)
  MATLAB Function9/1(k) -> Mux1/4
  MATLAB Function8/1(k) -> Mux1/3
  Constant6/1 -> MATLAB Function12/1(a)
  Constant1/1 -> MATLAB Function1/1(a)
  Constant8/1 -> MATLAB Function8/1(a)
  Constant3/1 -> MATLAB Function3/1(a)
  Constant2/1 -> MATLAB Function2/1(a)
  MATLAB Function5/1(k) -> Mux/6
  MATLAB Function4/1(k) -> Mux/5
  MATLAB Function11/1(k) -> Mux1/6
  Constant11/1 -> MATLAB Function11/1(a)
  MATLAB Function10/1(k) -> Mux1/5
  MATLAB Function7/1(k) -> Mux1/2
  Constant10/1 -> MATLAB Function10/1(a)
  Transpose/1 -> Product/1
  Transpose1/1 -> Product1/1
  MATLAB Function23/1(k) -> Mux4/3
  MATLAB Function15/1(k) -> Mux4/6
  Constant15/1 -> MATLAB Function15/1(a)
  Constant21/1 -> MATLAB Function22/1(a)
  Constant18/1 -> MATLAB Function19/1(a)
  Constant14/1 -> MATLAB Function14/1(a)
  MATLAB Function21/1(k) -> Mux2/1
  MATLAB Function14/1(k) -> Mux4/5
  MATLAB Function20/1(k) -> Mux2/6
  MATLAB Function16/1(k) -> Mux4/1
  MATLAB Function18/1(k) -> Mux2/4
  MATLAB Function17/1(k) -> Mux2/3
  Constant17/1 -> MATLAB Function18/1(a)
  Constant22/1 -> MATLAB Function23/1(a)
  Constant19/1 -> MATLAB Function20/1(a)
  Constant13/1 -> MATLAB Function13/1(a)
  Mux4/1 -> Transpose3/1
  MATLAB Function24/1(k) -> Mux4/4
  MATLAB Function19/1(k) -> Mux2/5
  Constant12/1 -> MATLAB Function21/1(a)
  Constant23/1 -> MATLAB Function24/1(a)
  Constant20/1 -> MATLAB Function16/1(a)
  Mux2/1 -> Transpose2/1
  Constant16/1 -> MATLAB Function17/1(a)
  length/1 -> MATLAB Function24/2(length), MATLAB Function14/2(length), MATLAB Function15/2(length), MATLAB Function23/2(length), MATLAB Function22/2(length), MATLAB Function16/2(length), MATLAB Function21/2(length), MATLAB Function13/2(length), MATLAB Function17/2(length), MATLAB Function18/2(length), MATLAB Function19/2(length), MATLAB Function20/2(length), MATLAB Function9/2(length), MATLAB Function10/2(length), MATLAB Function11/2(length), MATLAB Function8/2(length), MATLAB Function7/2(length), MATLAB Function12/2(length), MATLAB Function6/2(length), MATLAB Function1/2(length), MATLAB Function2/2(length), MATLAB Function3/2(length), MATLAB Function4/2(length), MATLAB Function5/2(length)
  MATLAB Function22/1(k) -> Mux4/2
  MATLAB Function13/1(k) -> Mux2/2
  Transpose2/1 -> Product2/1
  Transpose3/1 -> Product3/1
  Switch/1 -> T/1
  In7/1 -> Switch1/2, Switch/2
  Product/1 -> Switch/1
  Product2/1 -> Switch/3
  Switch1/1 -> Tp/1
  Product1/1 -> Switch1/1
  Product3/1 -> Switch1/3

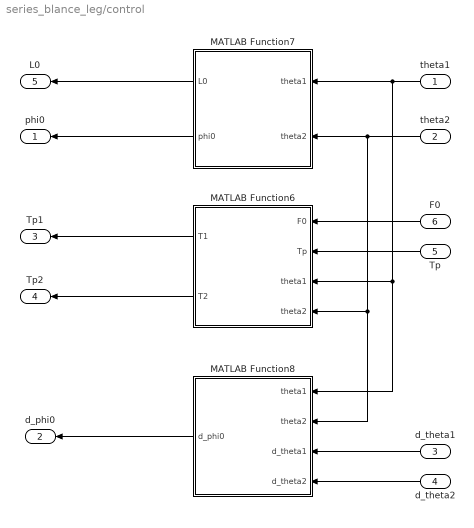
== system series_blance_leg/control ==
  theta1 : Inport
  theta2 : Inport  Port=2
  d_theta1 : Inport  Port=3
  d_theta2 : Inport  Port=4
  Tp : Inport  Port=5
  F0 : Inport  Port=6
  MATLAB Function6 : MATLAB Function  TreatAsAtomicUnit=on
  MATLAB Function7 : MATLAB Function  TreatAsAtomicUnit=on
  MATLAB Function8 : MATLAB Function  TreatAsAtomicUnit=on
  phi0 : Outport
  d_phi0 : Outport  Port=2
  Tp1 : Outport  Port=3
  Tp2 : Outport  Port=4
  L0 : Outport  Port=5
  wires:
  theta1/1 -> MATLAB Function8/1(theta1), MATLAB Function6/3(theta1), MATLAB Function7/1(theta1)
  theta2/1 -> MATLAB Function8/2(theta2), MATLAB Function6/4(theta2), MATLAB Function7/2(theta2)
  d_theta1/1 -> MATLAB Function8/3(d_theta1)
  d_theta2/1 -> MATLAB Function8/4(d_theta2)
  F0/1 -> MATLAB Function6/1(F0)
  Tp/1 -> MATLAB Function6/2(Tp)
  MATLAB Function7/1(L0) -> L0/1
  MATLAB Function7/2(phi0) -> phi0/1
  MATLAB Function6/1(T1) -> Tp1/1
  MATLAB Function6/2(T2) -> Tp2/1
  MATLAB Function8/1(d_phi0) -> d_phi0/1

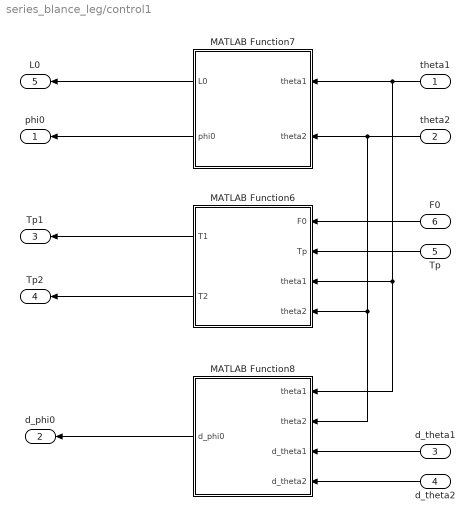
== system series_blance_leg/control1 ==
  theta1 : Inport
  theta2 : Inport  Port=2
  d_theta1 : Inport  Port=3
  d_theta2 : Inport  Port=4
  Tp : Inport  Port=5
  F0 : Inport  Port=6
  MATLAB Function6 : MATLAB Function  TreatAsAtomicUnit=on
  MATLAB Function7 : MATLAB Function  TreatAsAtomicUnit=on
  MATLAB Function8 : MATLAB Function  TreatAsAtomicUnit=on
  phi0 : Outport
  d_phi0 : Outport  Port=2
  Tp1 : Outport  Port=3
  Tp2 : Outport  Port=4
  L0 : Outport  Port=5
  wires:
  MATLAB Function8/1(d_phi0) -> d_phi0/1
  MATLAB Function6/2(T2) -> Tp2/1
  MATLAB Function6/1(T1) -> Tp1/1
  MATLAB Function7/2(phi0) -> phi0/1
  MATLAB Function7/1(L0) -> L0/1
  Tp/1 -> MATLAB Function6/2(Tp)
  F0/1 -> MATLAB Function6/1(F0)
  d_theta2/1 -> MATLAB Function8/4(d_theta2)
  d_theta1/1 -> MATLAB Function8/3(d_theta1)
  theta2/1 -> MATLAB Function7/2(theta2), MATLAB Function6/4(theta2), MATLAB Function8/2(theta2)
  theta1/1 -> MATLAB Function7/1(theta1), MATLAB Function6/3(theta1), MATLAB Function8/1(theta1)
